simulink library "commtimrec2"  (Simulink 6.0)
undefined symbols (not defined in the file or in its folder): D, i, magnitude
libraries: dspsigattribs x3, dspsigops x2, dspmtrx3 x1
settings Model: Creator=akansal  LastModifiedBy=akansal

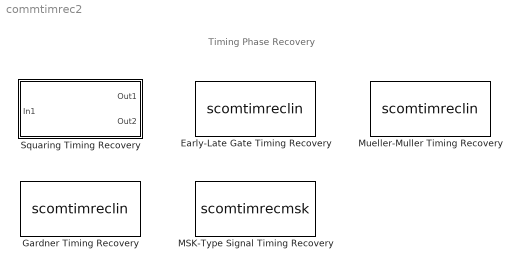
== system commtimrec2 ==
  note: Timing Phase Recovery
  Early-Late Gate Timing Recovery : S-Function  FunctionName=scomtimreclin  Parameters=sampPerSymbol, propGain, resetMode, 2  mask(Early-Late Gate Timing Recovery){sampPerSymbol=4, propGain=0.05, resetMode=None}
      mask prompts: sampPerSymbol "Samples per symbol:"; propGain "Error update gain:"; resetMode "Reset:"
      mask help:
      | Recover the symbol timing phase using the early-late gate method. This non-data-aided feedback method is suitable for linear baseband modulations.
      |
      | The method estimates the symbol timing phase offset for each incoming symbol and outputs the signal value corresponding to the estimated symbol sampling instant.
      |
      | The second output returns the estimated timing phase offset for each symbol, which is a nonnegative real number less than N where N is the number of samples per symbol.
      |
      | The error update gain parameter is the step size used for updating the successive phase estimates.
      mask init:
      | s = commblktimrec(resetMode);
      mask Help: helpview(commbhelp);
      mask StyleString: edit,edit,popup(None|Every frame|On nonzero input via port)
      mask Display:
      | disp('Early-Late Gate\nTiming Recovery');
      | port_label('input', s.i1, s.i1s);
      | port_label('input', s.i2, s.i2s);
      | port_label('output', s.o1, s.o1s);
      | port_label('output', s.o2, s.o2s);
  Gardner Timing Recovery : S-Function  FunctionName=scomtimreclin  Parameters=sampPerSymbol, propGain, resetMode, 1  mask(Gardner Timing Recovery){sampPerSymbol=4, propGain=0.05, resetMode=None}
      mask prompts: sampPerSymbol "Samples per symbol:"; propGain "Error update gain:"; resetMode "Reset:"
      mask help:
      | Recover the symbol timing phase using Gardner's method. This non-data-aided feedback method is suitable for linear baseband modulations.
      |
      | The method estimates the symbol timing phase offset for each incoming symbol and outputs the signal value corresponding to the estimated symbol sampling instant.
      |
      | The second output returns the estimated timing phase offset for each symbol, which is a nonnegative real number less than N where N is the number of samples per symbol.
      |
      | The error update gain parameter is the step size used for updating the successive phase estimates.
      mask init:
      | s = commblktimrec(resetMode);
      mask Help: helpview(commbhelp);
      mask StyleString: edit,edit,popup(None|Every frame|On nonzero input via port)
      mask Display:
      | disp('Gardner\nTiming Recovery');
      | port_label('input', s.i1, s.i1s);
      | port_label('input', s.i2, s.i2s);
      | port_label('output', s.o1, s.o1s);
      | port_label('output', s.o2, s.o2s);
  MSK-Type Signal Timing Recovery : S-Function  FunctionName=scomtimrecmsk  Parameters=sampPerSymbol, propGain, resetMode, modType  mask(MSK-Type Signal Timing Recovery){modType=MSK, sampPerSymbol=4, propGain=0.05, resetMode=None}
      mask prompts: modType "Modulation type:"; sampPerSymbol "Samples per symbol:"; propGain "Error update gain:"; resetMode "Reset:"
      mask help:
      | Recover the symbol timing phase using a fourth-order non-linearity method. This non-data-aided feedback method is suitable for MSK-type baseband modulations.
      |
      | The method estimates the symbol timing phase offset for each incoming symbol and outputs the signal value corresponding to the estimated symbol sampling instant.
      |
      | The second output returns the estimated timing phase offset for each symbol, which is a nonnegative real number less than N where N is the number of samples per symbol.
      |
      | The error update gain parameter is the step size used for updating the successive phase estimates.
      mask init:
      | s = commblktimrec(resetMode, modType);
      mask Help: helpview(commbhelp);
      mask StyleString: popup(MSK|GMSK),edit,edit,popup(None|Every frame|On nonzero input via port)
      mask Display:
      | disp([s.type ' Signal\nTiming Recovery']);
      | port_label('input', s.i1, s.i1s);
      | port_label('input', s.i2, s.i2s);
      | port_label('output', s.o1, s.o1s);
      | port_label('output', s.o2, s.o2s);
  Mueller-Muller Timing Recovery : S-Function  FunctionName=scomtimreclin  Parameters=sampPerSymbol, propGain, resetMode, 3  mask(Mueller-Muller Timing Recovery){sampPerSymbol=4, propGain=0.05, resetMode=None}
      mask prompts: sampPerSymbol "Samples per symbol:"; propGain "Error update gain:"; resetMode "Reset:"
      mask help:
      | Recover the symbol timing phase using the Mueller-Muller method. This decision-directed data-aided feedback method is suitable for linear binary baseband modulations.
      |
      | The method estimates the symbol timing phase offset for each incoming symbol and outputs the signal value corresponding to the estimated symbol sampling instant.
      |
      | The second output returns the estimated timing phase offset for each symbol, which is a nonnegative real number less than N where N is the number of samples per symbol.
      |
      | The error update gain parameter is the step size used for updating the successive phase estimates.
      mask init:
      | s = commblktimrec(resetMode);
      mask Help: helpview(commbhelp);
      mask StyleString: edit,edit,popup(None|Every frame|On nonzero input via port)
      mask Display:
      | disp('Mueller-Muller\nTiming Recovery');
      | port_label('input', s.i1, s.i1s);
      | port_label('input', s.i2, s.i2s);
      | port_label('output', s.o1, s.o1s);
      | port_label('output', s.o2, s.o2s);
  Squaring Timing Recovery : Subsystem  mask(Squaring Timing Recovery){numSymb=100, sampPerSymb=4}
      mask prompts: numSymb "Symbols per frame:"; sampPerSymb "Samples per symbol:"
      mask help:
      | Recover the symbol timing phase using a Squaring method. This frame-based feed-forward method is suitable for linear baseband modulations.
      |
      | The method estimates the symbol timing phase offset for a sequence of symbols and outputs the symbol spaced signal values by applying the estimate uniformly over the sequence of data.
      |
      | The symbol timing phase offset is assumed to remain constant for an observation interval equal to the number of symbols in each frame.
      |
      | The second output returns the estimated timing phase offset for the data sequence, which is a nonnegative real number less than N where N is the number of samples per symbol.
      mask init:
      | commblksqtimrec2(numSymb, sampPerSymb);
      settings: ErrorFcn=commblktimrecechk
      mask Help: helpview(commbhelp);
      mask Display:
      | disp('Squaring\nTiming Recovery');
      | port_label('output',1,'Sym');
      | port_label('output',2,'Ph');

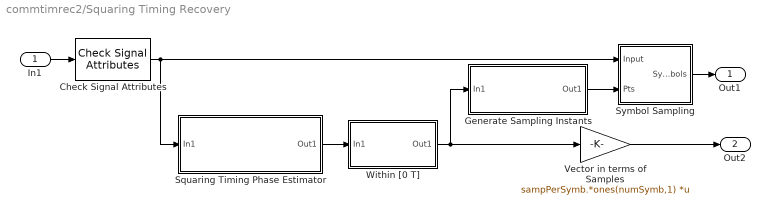
== system commtimrec2/Squaring Timing Recovery ==
  In1 : Inport
  Check Signal Attributes : dspsigattribs/Check Signal Attributes  SigAttribCheckMethod=Does not match attributes exactly  Complexity=Complex  Frame=Frame-based  DimsCheckMethod=Ignore  Dimensions=1-D  DatatypeCheckMethod=Ignore  DatatypeGeneral=Boolean  DtypeFloatSpecific=Any floating-point  DtypeFixedSpecific=Any fixed-point  DtypeIntSpecific=Any integer  SampleMode=Ignore
  Generate Sampling Instants : Subsystem  mask(Generate points){numSymb=numSymb, sampPerSymb=sampPerSymb}
      mask prompts: numSymb "Number of symbols:"; sampPerSymb "Samples per symbol:"
      mask help: Map the delay estimate to the symbol sampling instants for the number of symbols in the observation interval.
      mask Display:
      | disp('Generate\nInstants');
      | port_label('input',1,'Phase');
      | port_label('output',1,'Pts');
  Squaring Timing Phase Estimator : Subsystem  mask(Squaring Timing Phase Estimator ){obsInt=numSymb, L=sampPerSymb}
      mask prompts: obsInt "Observation interval (in symbols):"; L "Samples per symbol:"
      mask help:
      | A digital squaring timing phase estimator as proposed by Oerder and Meyr, this is a feed-forward method which uses the number of symbols as its observation interval to provide an estimate of the timing phase.
      |
      | The output timing phase estimate is in the interval [-T/2 T/2] where T is the normalized symbol period.
      |
      | The input frame length must be equal to the product of the observation interval length and the number of samples per symbol.
      mask Display:
      | disp('Squaring Timing\n Phase Estimator');
      | port_label('output',1,'Ph');
  Symbol Sampling : Subsystem
  Vector in terms of Samples : Gain  Gain=sampPerSymb.*ones(numSymb,1)  Multiplication=Matrix(K*u)  SaturateOnIntegerOverflow=on
  Within [0 T] : Subsystem  mask(Correct Interval ){threshold=(1/sampPerSymb)/2}
      mask help:
      | The block applies a threshold to the estimate input value and then converts the values [-T/2 T/2] to lie in the [0 T] range.
      |
      | If the absolute estimate is less than the threshold, it is set to 0. The threshold should be chosen less than 1/L where L is the number of samples per symbol.
      mask Display: disp('Correct\nInterval');
  Out1 : Outport
  Out2 : Outport  Port=2
  wires:
  Vector in terms of Samples/1 -> Out2/1
  Within [0 T]/1(Out1) -> Generate Sampling Instants/1(In1), Vector in terms of Samples/1
  Check Signal Attributes/1 -> Symbol Sampling/1(Input), Squaring Timing Phase Estimator/1(In1)
  Generate Sampling Instants/1(Out1) -> Symbol Sampling/2(Pts)
  Squaring Timing Phase Estimator/1(Out1) -> Within [0 T]/1(In1)
  Symbol Sampling/1(Symbols) -> Out1/1
  In1/1 -> Check Signal Attributes/1

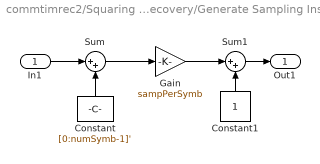
== system commtimrec2/Squaring Timing Recovery/Generate Sampling Instants ==
  In1 : Inport
  Constant : Constant  Orientation=up  Value=[0:numSymb-1]'
  Constant1 : Constant  Orientation=up
  Gain : Gain  Gain=sampPerSymb  SaturateOnIntegerOverflow=on
  Sum : Sum  Inputs=|++  SaturateOnIntegerOverflow=on
  Sum1 : Sum  Inputs=|++  SaturateOnIntegerOverflow=on
  Out1 : Outport
  wires:
  Sum1/1 -> Out1/1
  In1/1 -> Sum/1
  Gain/1 -> Sum1/1
  Constant1/1 -> Sum1/2
  Constant/1 -> Sum/2
  Sum/1 -> Gain/1

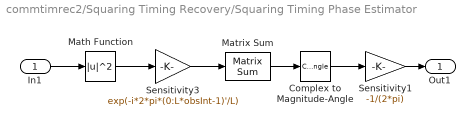
== system commtimrec2/Squaring Timing Recovery/Squaring Timing Phase Estimator ==
  In1 : Inport
  Complex to Magnitude-Angle : ComplexToMagnitudeAngle  Output=Angle
  Math Function : Math  Operator=magnitude^2  SaturateOnIntegerOverflow=on
  Matrix Sum : dspmtrx3/Matrix Sum  Dim=Columns  roundingMode=Floor  overflowMode=off
  Sensitivity1 : Gain  Gain=-1/(2*pi)  SaturateOnIntegerOverflow=on
  Sensitivity3 : Gain  Gain=exp(-i*2*pi*(0:L*obsInt-1)'/L)  SaturateOnIntegerOverflow=on
  Out1 : Outport
  wires:
  Math Function/1 -> Sensitivity3/1
  Matrix Sum/1 -> Complex to Magnitude-Angle/1
  Sensitivity3/1 -> Matrix Sum/1
  Complex to Magnitude-Angle/1 -> Sensitivity1/1
  In1/1 -> Math Function/1
  Sensitivity1/1 -> Out1/1

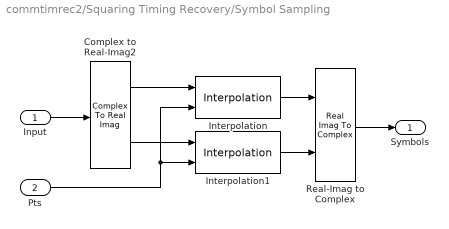
== system commtimrec2/Squaring Timing Recovery/Symbol Sampling ==
  Input : Inport
  Pts : Inport  Port=2
  Complex to Real-Imag2 : ComplexToRealImag
  Interpolation : dspsigops/Interpolation  InterpSource=Input port  InterpPoints=[1.1 4.8 2.67 1.6 3.2]'  InterpMode=Linear  InterpL=3  InterpR=3  InterpAlpha=0.5  InvalidMode=Clip
  Interpolation1 : dspsigops/Interpolation  InterpSource=Input port  InterpPoints=[1.1 4.8 2.67 1.6 3.2]'  InterpMode=Linear  InterpL=3  InterpR=3  InterpAlpha=0.5  InvalidMode=Clip
  Real-Imag to Complex : RealImagToComplex
  Symbols : Outport
  wires:
  Pts/1 -> Interpolation/2, Interpolation1/2
  Real-Imag to Complex/1 -> Symbols/1
  Input/1 -> Complex to Real-Imag2/1
  Interpolation1/1 -> Real-Imag to Complex/2
  Interpolation/1 -> Real-Imag to Complex/1
  Complex to Real-Imag2/2 -> Interpolation1/1
  Complex to Real-Imag2/1 -> Interpolation/1

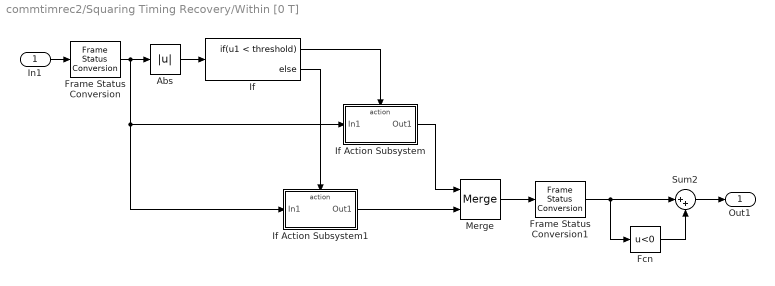
== system commtimrec2/Squaring Timing Recovery/Within [0 T] ==
  In1 : Inport
  Abs : Abs  SaturateOnIntegerOverflow=on
  Fcn : Fcn  Expr=u<0
  Frame Status Conversion : dspsigattribs/Frame Status Conversion  growRefPort=off  outframe=Sample-based
  Frame Status Conversion1 : dspsigattribs/Frame Status Conversion  growRefPort=off  outframe=Frame-based
  If : If  IfExpression=u1 < threshold
  If Action Subsystem : Subsystem  TreatAsAtomicUnit=on
  If Action Subsystem1 : Subsystem  AncestorBlock=commsyncprivate/Subsystem/If Action Subsystem  TreatAsAtomicUnit=on
  Merge : Merge
  Sum2 : Sum  Inputs=|++  SaturateOnIntegerOverflow=on
  Out1 : Outport
  wires:
  Sum2/1 -> Out1/1
  Frame Status Conversion1/1 -> Fcn/1, Sum2/1
  Fcn/1 -> Sum2/2
  Abs/1 -> If/1
  Frame Status Conversion/1 -> Abs/1, If Action Subsystem/1(In1), If Action Subsystem1/1(In1)
  If/1 -> If Action Subsystem/Action
  In1/1 -> Frame Status Conversion/1
  If/2 -> If Action Subsystem1/Action
  If Action Subsystem1/1(Out1) -> Merge/2
  If Action Subsystem/1(Out1) -> Merge/1
  Merge/1 -> Frame Status Conversion1/1

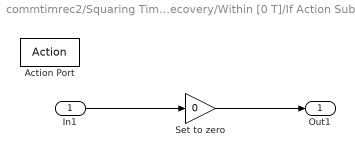
== system commtimrec2/Squaring Timing Recovery/Within [0 T]/If Action Subsystem ==
  In1 : Inport
  Action Port : ActionPort
  Set to zero : Gain  Gain=0  SaturateOnIntegerOverflow=on
  Out1 : Outport
  wires:
  Set to zero/1 -> Out1/1
  In1/1 -> Set to zero/1

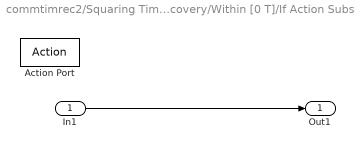
== system commtimrec2/Squaring Timing Recovery/Within [0 T]/If Action Subsystem1 ==
  In1 : Inport
  Action Port : ActionPort
  Out1 : Outport
  wires:
  In1/1 -> Out1/1
